simulink model "regolatore_manipolatore"  (R2024b)
settings: Solver=VariableStepAuto  StartTime=0.0  StopTime=100  RelTol=1e-3
values from neighbouring files (symbols this model uses):
  kd = K(:,3:4)    [regolatore_robot.m]
  kp = K(:,1:2)    [regolatore_robot.m]
settings Model: Creator=Davide  LastModifiedBy=david
settings OptimizationCC: ReuseModelBlockBuffer=off
settings RTWCC: GPUComputeCapability=3.5

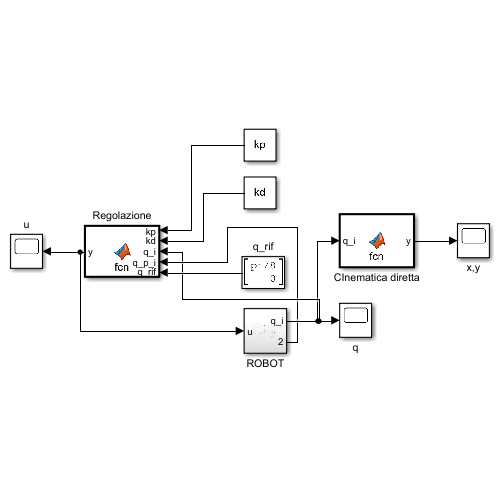
[thumbnail: Simulink's stored preview of the top-level diagram]
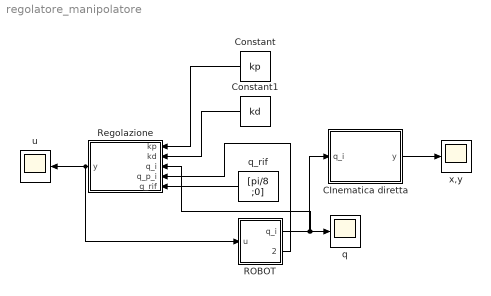
== system regolatore_manipolatore ==
  CInematica diretta : MATLAB Function  TreatAsAtomicUnit=on
  Constant : Constant  Value=kp  VectorParams1D=off
  Constant1 : Constant  Value=kd  VectorParams1D=off
  ROBOT : Subsystem
  Regolazione : MATLAB Function  TreatAsAtomicUnit=on
  q : Scope
  q_rif : Constant  Value=[pi/8 ;0]  VectorParams1D=off
  u : Scope
  x,y : Scope
  wires:
  Regolazione/1(y) -> u/1, ROBOT/1(u)
  CInematica diretta/1(y) -> x,y/1
  q_rif/1 -> Regolazione/5(q_rif)
  Constant/1 -> Regolazione/1(kp)
  Constant1/1 -> Regolazione/2(kd)
  ROBOT/2(Out2) -> Regolazione/4(q_p_i)
  ROBOT/1(q_i) -> Regolazione/3(q_i), q/1, CInematica diretta/1(q_i)

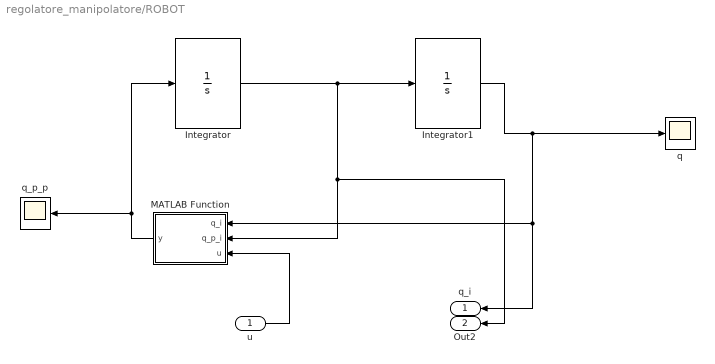
== system regolatore_manipolatore/ROBOT ==
  u : Inport
  Integrator : Integrator  InitialCondition=[0;0]
  Integrator1 : Integrator  InitialCondition=[0;0]
  MATLAB Function : MATLAB Function  TreatAsAtomicUnit=on
  q : Scope
  q_p_p : Scope
  q_i : Outport
  Out2 : Outport  Port=2
  wires:
  u/1 -> MATLAB Function/3(u)
  Integrator/1 -> Out2/1, MATLAB Function/2(q_p_i), Integrator1/1
  MATLAB Function/1(y) -> Integrator/1, q_p_p/1
  Integrator1/1 -> q_i/1, MATLAB Function/1(q_i), q/1

== matlab function regolatore_manipolatore/ROBOT/MATLAB Function ==
  data: q_i input; q_p_i input; u input; y output
function y = fcn(q_i,q_p_i,u)


theta1 = 10.6125; 
theta2 = 0.85; 
theta3 = 2.25;
theta4 = 1.6;
theta5 = 80.9325;
theta6 = 14.7150;
q = q_i;
q_p = q_p_i;
v = u;
F1 = 15;
F2 = 10;

B = [theta1 + 2*theta3*q(2) theta2+theta3*cos(q(2)) ; ...
     theta2+theta3*cos(q(2)) theta4];
C = [-2*theta3*q_p(2)*sin(q(2))  -theta3*q_p(2)*sin(q(2)) ; ...
      theta3*q_p(1)*sin(q(2))              0              ];
g = [theta5*cos(q(1))+theta6*cos(q(1)+q(2)) ; theta6*cos(q(1)+q(2))];
F = [F1*q_p(1) ; F2*q_p(2)];

y = inv(B)*(v - g - F - C*q_p);

== matlab function regolatore_manipolatore/Regolazione ==
  data: kp input; kd input; q_i input; q_p_i input; q_rif input; y output
function y = fcn(kp,kd,q_i,q_p_i,q_rif)


theta5 = 80.9325;
theta6 = 14.7150;
q = q_i;
q_p = q_p_i;
q_r = q_rif;

g = [theta5*cos(q(1))+theta6*cos(q(1)+q(2)) ; theta6*cos(q(1)+q(2))];


y = g - kp*(q-q_r) - kd*q_p;

== matlab function regolatore_manipolatore/CInematica diretta ==
  data: q_i input; y output
function y = fcn(q_i)

q = q_i;
l1 = 1.5;
l2 = 1;

%Estrazione posizione spazio operativo
y = [l1*cos(q(1))+l2*cos(q(2)) ; l1*sin(q(1))+l2*sin(q(2))];
